simulink model "stiffnessTrace"  (R2018a)
settings: Solver=FixedStepAuto  StartTime=0.0  StopTime=10.0  FixedStep=0.01  RelTol=1e-3
libraries: simulink x1
settings Model: Creator=pei-T  LastModifiedBy=pei-T

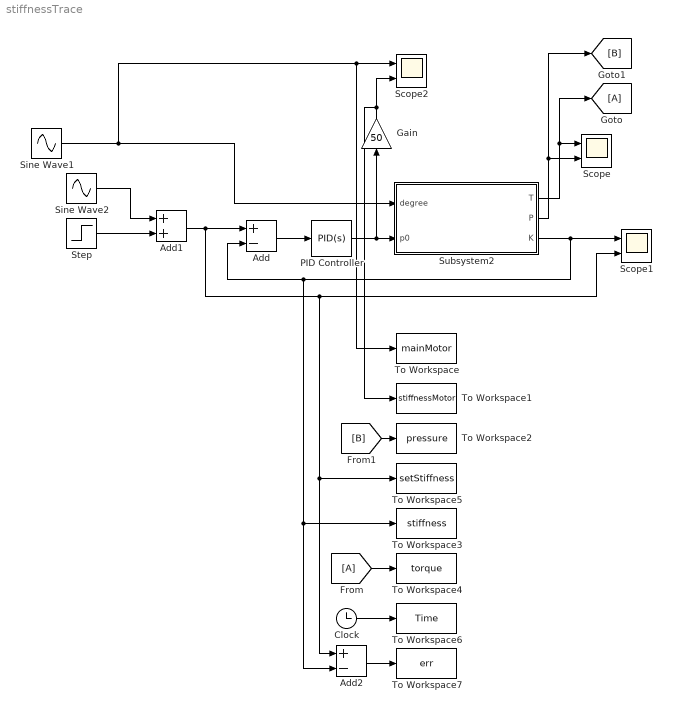
== system stiffnessTrace ==
  Add : Sum  Inputs=+-
  Add1 : Sum
  Add2 : Sum  Inputs=+-
  Clock : Clock
  Gain : Gain  Gain=50
  PID Controller : simulink/Continuous/PID Controller  Controller=PID  TimeDomain=Continuous-time  SampleTime=-1  IntegratorMethod=Forward Euler  FilterMethod=Forward Euler  Form=Parallel  UseFilter=on  ControllerParametersSource=internal  P=0  I=117.676591343019  D=0  N=100  InitialConditionSource=internal  InitialConditionForIntegrator=0  InitialConditionForFilter=0  ExternalReset=none  LimitOutput=on  UpperSaturationLimit=0.8  LowerSaturationLimit=0  LinearizeAsGain=on  AntiWindupMode=none  Kb=1  TrackingMode=off  Kt=1  PParamMin=[]  PParamMax=[]  IParamMin=[]  IParamMax=[]  DParamMin=[]  DParamMax=[]  NParamMin=[]  NParamMax=[]  KbParamMin=[]  KbParamMax=[]  KtParamMin=[]  KtParamMax=[]  POutMin=[]  POutMax=[]  IOutMin=[]  IOutMax=[]  DOutMin=[]  DOutMax=[]  NOutMin=[]  NOutMax=[]  KbOutMin=[]  KbOutMax=[]  KtOutMin=[]  KtOutMax=[]  IntegratorOutMin=[]  IntegratorOutMax=[]  FilterOutMin=[]  FilterOutMax=[]  SumOutMin=[]  SumOutMax=[]  SumI1OutMin=[]  SumI1OutMax=[]  SumI2OutMin=[]  SumI2OutMax=[]  SumI3OutMin=[]  SumI3OutMax=[]  SumDOutMin=[]  SumDOutMax=[]  SaturationOutMin=[]  SaturationOutMax=[]  IntegratorContinuousStateAttributes=''  IntegratorStateMustResolveToSignalObject=off  IntegratorRTWStateStorageClass=Auto  FilterContinuousStateAttributes=''  FilterStateMustResolveToSignalObject=off  FilterRTWStateStorageClass=Auto  DifferentiatorICPrevScaledInput=0  DifferentiatorOutMin=[]  DifferentiatorOutMax=[]  FilterDiffOutCoefMin=[]  FilterDiffOutCoefMax=[]  SumDenOutMin=[]  SumDenOutMax=[]  SumNumOutMin=[]  SumNumOutMax=[]  ReciprocalOutMin=[]  ReciprocalOutMax=[]  DivideOutMin=[]  DivideOutMax=[]  TunerSelectOption=Transfer Function Based (PID Tuner App)
  Scope : Scope  NumInputPorts=2
  Scope1 : Scope  NumInputPorts=2
  Scope2 : Scope  NumInputPorts=2
  Sine Wave1 : Sin  Amplitude=30  SampleTime=0
  Sine Wave2 : Sin  Amplitude=0.01  SampleTime=0
  Step : Step  Time=0  After=0.05  SampleTime=0
  Subsystem2 : Subsystem
  To Workspace : ToWorkspace  VariableName=mainMotor  SampleTime=-1
      settings: Save2DSignal=2-D array (concatenate along first dimension)
  To Workspace1 : ToWorkspace  VariableName=stiffnessMotor  SampleTime=-1
      settings: Save2DSignal=2-D array (concatenate along first dimension)
  To Workspace2 : ToWorkspace  VariableName=pressure  SampleTime=-1
      settings: Save2DSignal=2-D array (concatenate along first dimension)
  To Workspace3 : ToWorkspace  VariableName=stiffness  SampleTime=-1
      settings: Save2DSignal=2-D array (concatenate along first dimension)
  To Workspace4 : ToWorkspace  VariableName=torque  SampleTime=-1
      settings: Save2DSignal=2-D array (concatenate along first dimension)
  To Workspace5 : ToWorkspace  VariableName=setStiffness  SampleTime=-1
      settings: Save2DSignal=2-D array (concatenate along first dimension)
  To Workspace6 : ToWorkspace  VariableName=Time  SampleTime=-1
      settings: Save2DSignal=2-D array (concatenate along first dimension)
  To Workspace7 : ToWorkspace  VariableName=err  SampleTime=-1
      settings: Save2DSignal=2-D array (concatenate along first dimension)
  wires:
  Sine Wave1/1 -> To Workspace/1, Scope2/1, Subsystem2/1(degree)
  Subsystem2/1(T) -> [A], Scope/1
  Subsystem2/3(K) -> Add2/2, To Workspace3/1, Add/2, Scope1/1
  Add/1 -> PID Controller/1
  Add1/1 -> Add2/1, To Workspace5/1, Scope1/2, Add/1
  PID Controller/1 -> Gain/1, Subsystem2/2(p0)
  Sine Wave2/1 -> Add1/1
  Step/1 -> Add1/2
  Subsystem2/2(P) -> [B], Scope/2
  Gain/1 -> To Workspace1/1, Scope2/2
  [A] -> To Workspace4/1
  [B] -> To Workspace2/1
  Clock/1 -> To Workspace6/1
  Add2/1 -> To Workspace7/1

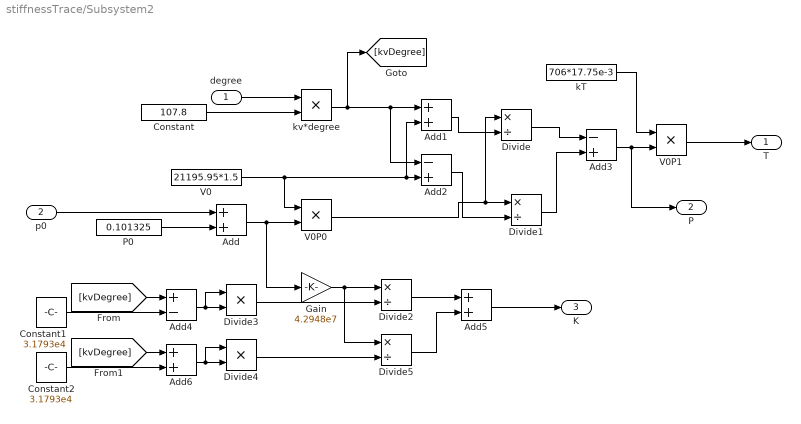
== system stiffnessTrace/Subsystem2 ==
  degree : Inport
  p0 : Inport  Port=2
  Add{,1,5..6} (4 alike) : Sum
  Add2 : Sum  Inputs=-+
  Add3 : Sum  Inputs=-+
  Add4 : Sum  Inputs=+-
  Constant : Constant  Value=107.8
  Constant1 : Constant  Value=3.1793e4
  Constant2 : Constant  Value=3.1793e4
  Divide{,1..2,5} (4 alike) : Product  Inputs=*/
  Divide3 : Product  Inputs=**
  Divide4 : Product  Inputs=**
  Gain : Gain  Gain=4.2948e7
  P0 : Constant  Value=0.101325
  V0 : Constant  Value=21195.95*1.5
  V0P0 : Product
  V0P1 : Product
  kT : Constant  Value=706*17.75e-3
  kv*degree : Product
  T : Outport
  P : Outport  Port=2
  K : Outport  Port=3
  wires:
  Add3/1 -> P/1, V0P1/2
  V0/1 -> V0P0/1, Add2/2, Add1/2
  V0P1/1 -> T/1
  p0/1 -> Add/1
  Constant/1 -> kv*degree/2
  degree/1 -> kv*degree/1
  Add/1 -> Gain/1, V0P0/2
  P0/1 -> Add/2
  kv*degree/1 -> [kvDegree], Add2/1, Add1/1
  kT/1 -> V0P1/1
  V0P0/1 -> Divide1/1, Divide/1
  Add2/1 -> Divide1/2
  Add1/1 -> Divide/2
  Divide1/1 -> Add3/2
  Divide/1 -> Add3/1
  Gain/1 -> Divide5/1, Divide2/1
  [kvDegree] -> Add4/1
  Constant1/1 -> Add4/2
  Add4/1 -> Divide3/1, Divide3/2
  Divide3/1 -> Divide2/2
  Divide2/1 -> Add5/1
  Add6/1 -> Divide4/1, Divide4/2
  [kvDegree] -> Add6/1
  Constant2/1 -> Add6/2
  Divide4/1 -> Divide5/2
  Divide5/1 -> Add5/2
  Add5/1 -> K/1
